simulink model "Laboratorio_grupal_v6_R2024b"  (R2024b)
settings: Solver=ode4  StartTime=0.0  StopTime=8  FixedStep=0.01  RelTol=1e-3
model workspace (MATLAB code in the model file):
  | % Definición de constantes
  | K = 0.28;         % 1/hora
  | k12 = 1.78;       % 1/hora
  | k21 = 2.20;       % 1/hora
  | Ka = 1.80;        % 1/hora
  | ke1 = 0.83;       % 1/hora
  | ke0 = 0.83;       % 1/hora
  | F = 0.89;         % Litro/hora
  | Emax = 5.17;      % Sin unidad
  | EC50 = 9.98;      % mg/Litro
  | Cgut_0=200;       % mg/Litro
  | C1_0=1000;        % mg/Litro
  | C2_0=0;           % mg/Litro
  | Ce_0=0;           % mg/Litro
  | E0 = 10;          % Efecto basal
  | n=1;              %Pendiente de la curva
settings Model: Creator=Lucia  LastModifiedBy=MyJ
settings RTWCC: GPUComputeCapability=3.5

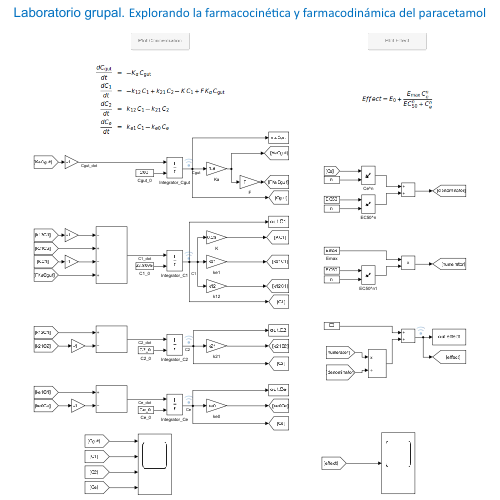
[thumbnail: Simulink's stored preview of the top-level diagram]
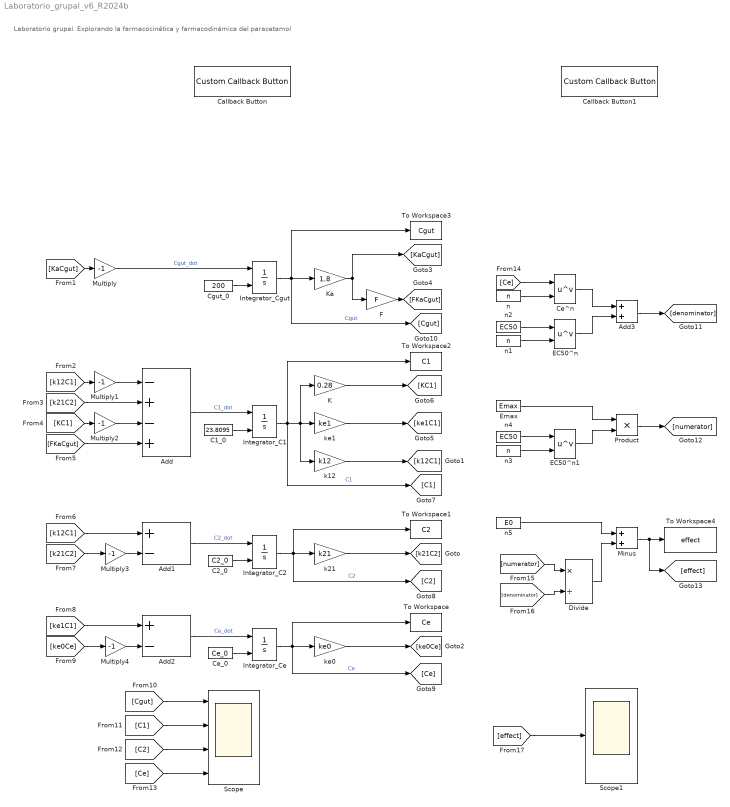
== system Laboratorio_grupal_v6_R2024b ==
  note: Laboratorio grupal. Explorando la farmacocinética y farmacodinámica del paracetamol
  Add : Sum  Inputs=-+-+
  Add1 : Sum  Inputs=+-
  Add2 : Sum  Inputs=+-
  Add3 : Sum
  C1_0 : Constant  Value=23.8095
  C2_0 : Constant  Value=C2_0
  Callback Button : CustomCallbackButton  Configuration="{\"components\":[{\"name\":\"BackgroundImageComponent\",\"settings\":{\"image\":{\"size\":[0,0],\"src\":\"default\",\"srcOrientation\":\"Right\"},\"position\":[0,0,1,1]}},{\"name\":\"ButtonStateComponent\",\"settings\":{\"buttonType\":\"momentary\",\"clickFcn\":\"%Plots\\n% Crear los subplots\\nfigure;\\n\\n% Subplot 1: Concentración en el intestino (Cgut)\\nsubplot(4,1,1);\\nplot(Cgut.Time, Cgut.Data, 'LineWidth', 1.5);\\ntitle('Concentración en el Intestino (Cgut)');\\nxlabel('Tiempo (s)');\\nylabel('Concentración');\\ngrid on;\\n\\n% Subplot 2: Concentración en el compartimento 1 (C1)\\nsubplot(4,1,2);\\nplot(C1.Time, C1.Data, 'LineWidth', 1.5);\\ntitle('Concentración en el Compartimento 1 (C1)');\\nxlabel('Tiempo (s)');\\nylabel('Concentración');\\ngrid on;\\n\\n% Subplot 3: Concentración en el compartimento 2 (C2)\\nsubplot(4,1,3);\\nplot(C2.Time, C2.Data, 'LineWidth', 1.5);\\ntitle('Concentración en el Compartimento 2 (C2)');\\nxlabel('Tiempo (s)');\\nylabel('Concentración');\\ngrid on;\\n\\n% Subplot 4: Concentración en el efecto (Ce)\\nsubplot(4,1,4);\\nplot(Ce.Time, Ce.Data, 'LineWidth', 1.5);\\ntitle('Concentración en el Efecto (Ce)');\\nxlabel('Tiempo (s)');\\nylabel('Concentración');\\ngrid on;\",\"onValue\":1,\"position\":[0,0,1,1],\"pressDelay\":\"500\",\"pressFcn\":\"\",\"repeatInterval\":\"0\",\"states\":[{\"horizontalAlignment\":\"center\",\"image\":{\"position\":[0,0,1,1],\"size\":[1,1],\"src\":\"default\",\"srcOrientation\":\"Right\"},\"label\":{\"color\":[0.01176470588,0.01176470588,0.01176470588,1],\"icon\":{\"size\":[0,0],\"src\":\"default\",\"srcOrientation\":\"Right\"},\"iconPlacement\":\"left\",\"opacity\":1,\"show\":true,\"text\":{\"content\":\"Plot Concentration\",\"font\":\"Helvetica\"}},\"labelOffset\":[0,0],\"verticalAlignment\":\"middle\"},{\"horizontalAlignment\":\"center\",\"image\":{\"position\":[0,0,1,1],\"size\":[1,1],\"src\":\"default\",\"srcOrientation\":\"Right\"},\"label\":{\"color\":[0.01176470588,0.01176470588,0.01176470588,1],\"icon\":{\"size\":[0,0],\"src\":\"default\",\"srcOrientation\":\"Right\"},\"iconPlacement\":\"left\",\"opacity\":1,\"show\":true,\"text\":{\"content\":\"Plot Concentration\",\"font\":\"Helvetica\"}},\"labelOffset\":[0,0],\"verticalAlignment\":\"middle\"},{\"horizontalAlignment\":\"center\",\"image\":{\"position\":[0,0,1,1],\"size\":[1,1],\"src\":\"default\",\"srcOrientation\":\"Right\"},\"label\":{\"color\":[0.01176470588,0.01176470588,0.01176470588,1],\"icon\":{\"size\":[0,0],\"src\":\"default\",\"srcOrientation\":\"Right\"},\"iconPlacement\":\"left\",\"opacity\":1,\"show\":true,\"text\":{\"content\":\"Plot Concentration\",\"font\":\"Helvetica\"}},\"labelOffset\":[0,0],\"verticalAlignment\":\"middle\"},{\"horizontalAlignment\":\"center\",\"image\":{\"position\":[0,0,1,1],\"size\":[1,1],\"src\":\"default\",\"srcOrientation\":\"Right\"},\"label\":{\"color\":[0.01176470588,0.01176470588,0.01176470588,1],\"icon\":{\"size\":[0,0],\"src\":\"default\",\"srcOrientation\":\"Right\"},\"iconPlacement\":\"left\",\"opacity\":1,\"show\":true,\"text\":{\"content\":\"Plot Concentration\",\"font\":\"Helvetica\"}},\"labelOffset\":[0,0],\"verticalAlignment\":\"middle\"}]}},{\"name\":\"ForegroundImageComponent\",\"settings\":{\"image\":{\"size\":[0,0],\"src\":\"default\",\"srcOrientation\":\"Right\"},\"isForeground\":1,\"position\":[0,0,1,1]}}],\"settings\":{\"BindingType\":\"standalone\",\"backgroundColor\":[244,244,244,1],\"backgroundOffset\":0.2,\"backgroundOpacity\":1,\"fixedAspectRatio\":\"off\",\"foregroundColor\":[0.01176470588,0.01176470588,0.01176470588,1],\"migratedFromLegacy\":true,\"useBackgroundColor\":true,\"variant\":\"callback\",\"version\":\"R2024b\"},\"type\":\"Button\"}"  CustomBackgroundColor="{\"color\":[0.9568627451,0.9568627451,0.9568627451],\"show\":true}"
  Callback Button1 : CustomCallbackButton  Configuration="{\"components\":[{\"name\":\"BackgroundImageComponent\",\"settings\":{\"image\":{\"size\":[0,0],\"src\":\"default\",\"srcOrientation\":\"Right\"},\"position\":[0,0,1,1]}},{\"name\":\"ButtonStateComponent\",\"settings\":{\"buttonType\":\"momentary\",\"clickFcn\":\"%Plots\\n% Crear los subplots\\nfigure;\\n\\nplot(effect.Time, effect.Data, 'LineWidth', 1.5);\\ntitle('Efecto del fármaco (Effect)');\\nxlabel('Tiempo (h)');\\nylabel('Efecto');\\ngrid on;\\n\",\"onValue\":1,\"position\":[0,0,1,1],\"pressDelay\":\"500\",\"pressFcn\":\"\",\"repeatInterval\":\"0\",\"states\":[{\"horizontalAlignment\":\"center\",\"image\":{\"position\":[0,0,1,1],\"size\":[1,1],\"src\":\"default\",\"srcOrientation\":\"Right\"},\"label\":{\"color\":[0.01176470588,0.01176470588,0.01176470588,1],\"icon\":{\"size\":[0,0],\"src\":\"default\",\"srcOrientation\":\"Right\"},\"iconPlacement\":\"left\",\"opacity\":1,\"show\":true,\"text\":{\"content\":\"Plot Effect\",\"font\":\"Helvetica\"}},\"labelOffset\":[0,0],\"verticalAlignment\":\"middle\"},{\"horizontalAlignment\":\"center\",\"image\":{\"position\":[0,0,1,1],\"size\":[1,1],\"src\":\"default\",\"srcOrientation\":\"Right\"},\"label\":{\"color\":[0.01176470588,0.01176470588,0.01176470588,1],\"icon\":{\"size\":[0,0],\"src\":\"default\",\"srcOrientation\":\"Right\"},\"iconPlacement\":\"left\",\"opacity\":1,\"show\":true,\"text\":{\"content\":\"Plot Effect\",\"font\":\"Helvetica\"}},\"labelOffset\":[0,0],\"verticalAlignment\":\"middle\"},{\"horizontalAlignment\":\"center\",\"image\":{\"position\":[0,0,1,1],\"size\":[1,1],\"src\":\"default\",\"srcOrientation\":\"Right\"},\"label\":{\"color\":[0.01176470588,0.01176470588,0.01176470588,1],\"icon\":{\"size\":[0,0],\"src\":\"default\",\"srcOrientation\":\"Right\"},\"iconPlacement\":\"left\",\"opacity\":1,\"show\":true,\"text\":{\"content\":\"Plot Effect\",\"font\":\"Helvetica\"}},\"labelOffset\":[0,0],\"verticalAlignment\":\"middle\"},{\"horizontalAlignment\":\"center\",\"image\":{\"position\":[0,0,1,1],\"size\":[1,1],\"src\":\"default\",\"srcOrientation\":\"Right\"},\"label\":{\"color\":[0.01176470588,0.01176470588,0.01176470588,1],\"icon\":{\"size\":[0,0],\"src\":\"default\",\"srcOrientation\":\"Right\"},\"iconPlacement\":\"left\",\"opacity\":1,\"show\":true,\"text\":{\"content\":\"Plot Effect\",\"font\":\"Helvetica\"}},\"labelOffset\":[0,0],\"verticalAlignment\":\"middle\"}]}},{\"name\":\"ForegroundImageComponent\",\"settings\":{\"image\":{\"size\":[0,0],\"src\":\"default\",\"srcOrientation\":\"Right\"},\"isForeground\":1,\"position\":[0,0,1,1]}}],\"settings\":{\"BindingType\":\"standalone\",\"backgroundColor\":[244,244,244,1],\"backgroundOffset\":0.2,\"backgroundOpacity\":1,\"fixedAspectRatio\":\"off\",\"foregroundColor\":[0.01176470588,0.01176470588,0.01176470588,1],\"migratedFromLegacy\":true,\"useBackgroundColor\":true,\"variant\":\"callback\",\"version\":\"R2024b\"},\"type\":\"Button\"}"  CustomBackgroundColor="{\"color\":[0.9568627451,0.9568627451,0.9568627451],\"show\":true}"
  Ce^n : Math  Operator=pow
  Ce_0 : Constant  Value=Ce_0
  Cgut_0 : Constant  Value=200
  Divide : Product  Inputs=*/
  EC50^n : Math  Operator=pow
  EC50^n1 : Math  Operator=pow
  Emax : Constant  Value=Emax
  F : Gain  Gain=F
  Integrator_C1 : Integrator  InitialConditionSource=external
  Integrator_C2 : Integrator  InitialConditionSource=external
  Integrator_Ce : Integrator  InitialConditionSource=external
  Integrator_Cgut : Integrator  InitialConditionSource=external
  K : Gain  Gain=0.28
  Ka : Gain  Gain=1.8
  Minus : Sum
  Multiply{,1..4} (5 alike) : Gain  Gain=-1
  Product : Product
  Scope : Scope  NumInputPorts=4
  Scope1 : Scope
  To Workspace : ToWorkspace  VariableName=Ce  SaveFormat=Timeseries  SampleTime=-1
  To Workspace1 : ToWorkspace  VariableName=C2  SaveFormat=Timeseries  SampleTime=-1
  To Workspace2 : ToWorkspace  VariableName=C1  SaveFormat=Timeseries  SampleTime=-1
  To Workspace3 : ToWorkspace  VariableName=Cgut  SaveFormat=Timeseries  SampleTime=-1
  To Workspace4 : ToWorkspace  VariableName=effect  SaveFormat=Timeseries  SampleTime=-1
  k12 : Gain  Gain=k12
  k21 : Gain  Gain=k21
  ke0 : Gain  Gain=ke0
  ke1 : Gain  Gain=ke1
  n : Constant  Value=n
  n1 : Constant  Value=n
  n2 : Constant  Value=EC50
  n3 : Constant  Value=n
  n4 : Constant  Value=EC50
  n5 : Constant  Value=E0
  wires:
  Integrator_C1/1 -> [C1], To Workspace2/1, k12/1, K/1, ke1/1  "C1"
  k21/1 -> [k21C2]
  k12/1 -> [k12C1]
  Integrator_Ce/1 -> [Ce], To Workspace/1, ke0/1  "Ce"
  ke0/1 -> [ke0Ce]
  Integrator_Cgut/1 -> [Cgut], To Workspace3/1, Ka/1  "Cgut"
  Ka/1 -> F/1, [KaCgut]
  ke1/1 -> [ke1C1]
  K/1 -> [KC1]
  F/1 -> [FKaCgut]
  [KaCgut] -> Multiply/1
  [k12C1] -> Multiply1/1
  Multiply1/1 -> Add/1
  [k21C2] -> Add/2
  [KC1] -> Multiply2/1
  Multiply2/1 -> Add/3
  [FKaCgut] -> Add/4
  Add/1 -> Integrator_C1/1  "C1_dot"
  [k12C1] -> Add1/1
  Multiply3/1 -> Add1/2
  [k21C2] -> Multiply3/1
  Add1/1 -> Integrator_C2/1  "C2_dot"
  [ke0Ce] -> Multiply4/1
  [ke1C1] -> Add2/1
  Multiply4/1 -> Add2/2
  C1_0/1 -> Integrator_C1/2
  Integrator_C2/1 -> [C2], To Workspace1/1, k21/1  "C2"
  Add2/1 -> Integrator_Ce/1  "Ce_dot"
  Multiply/1 -> Integrator_Cgut/1  "Cgut_dot"
  Cgut_0/1 -> Integrator_Cgut/2
  C2_0/1 -> Integrator_C2/2
  Ce_0/1 -> Integrator_Ce/2
  [Cgut] -> Scope/1
  [C1] -> Scope/2
  [C2] -> Scope/3
  [Ce] -> Scope/4
  [Ce] -> Ce^n/1
  n/1 -> Ce^n/2
  n2/1 -> EC50^n/1
  n1/1 -> EC50^n/2
  Ce^n/1 -> Add3/1
  EC50^n/1 -> Add3/2
  Add3/1 -> [denominator]
  Emax/1 -> Product/1
  n4/1 -> EC50^n1/1
  n3/1 -> EC50^n1/2
  EC50^n1/1 -> Product/2
  Product/1 -> [numerator]
  n5/1 -> Minus/1
  [numerator] -> Divide/1
  [denominator] -> Divide/2
  Divide/1 -> Minus/2
  Minus/1 -> [effect], To Workspace4/1
  [effect] -> Scope1/1
